simulink model "Nodal_Analysis"  (R2024b)
settings: Solver=VariableStepAuto  StartTime=0.0  StopTime=10.0  RelTol=1e-3
libraries: spsSeriesRLCBranchLib x15, spsVoltageMeasurementLib x13, spsDCVoltageSourceLib x5, spsACVoltageSourceLib x2, spsCurrentMeasurementLib x1, spsControlledCurrentSourceLib x1, sps_lib x1
settings Model: Creator=priya  LastModifiedBy=priya

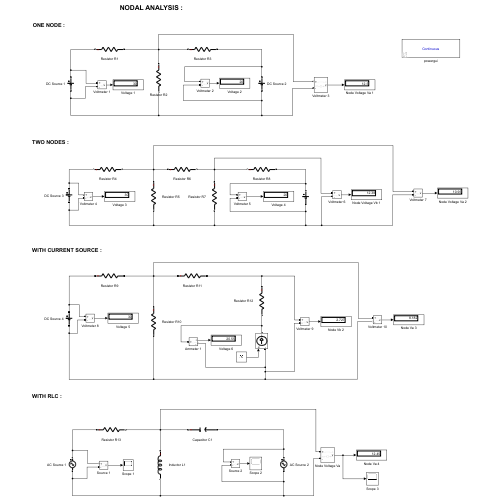
[thumbnail: Simulink's stored preview of the top-level diagram]
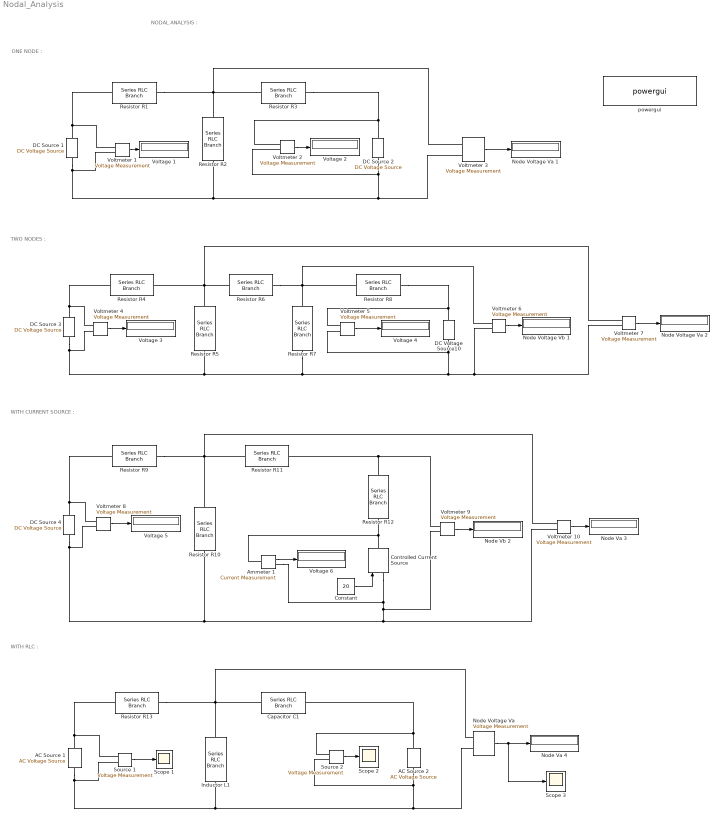
== system Nodal_Analysis ==
  note: WITH CURRENT SOURCE :
  note: TWO NODES :
  note: ONE NODE :
  note: NODAL ANALYSIS :
  note: WITH RLC :
  AC Source 1 : spsACVoltageSourceLib/AC Voltage Source  Amplitude=30  Phase=0  Frequency=60  SampleTime=0  Measurements=None  BusType=swing  Pref=10e3  Qref=0  Qmin=-inf  Qmax=+inf
  AC Source 2 : spsACVoltageSourceLib/AC Voltage Source  Amplitude=20  Phase=0  Frequency=60  SampleTime=0  Measurements=None  BusType=swing  Pref=10e3  Qref=0  Qmin=-inf  Qmax=+inf
  Ammeter 1 : spsCurrentMeasurementLib/Current Measurement  PhasorSimulation=off  OutputType=Complex  PSBequivalent=0
  Capacitor C1 : spsSeriesRLCBranchLib/Series RLC Branch  LConnTagsString=__new0  RConnTagsString=__new0  BranchType=C  Resistance=10  Inductance=1e-3  SetiL0=off  InitialCurrent=0  Capacitance=106.1e-6  Setx0=off  InitialVoltage=0  Measurements=None
  Constant : Constant  Value=20
  Controlled Current Source : spsControlledCurrentSourceLib/Controlled Current Source  Initialize=on  Source_Type=DC  Amplitude=20  Phase=0  Frequency=0  Measurements=None
  DC Source 1 : spsDCVoltageSourceLib/DC Voltage Source  Amplitude=30  Measurements=None
  DC Source 2 : spsDCVoltageSourceLib/DC Voltage Source  Amplitude=20  Measurements=None
  DC Source 3 : spsDCVoltageSourceLib/DC Voltage Source  Amplitude=30  Measurements=None
  DC Source 4 : spsDCVoltageSourceLib/DC Voltage Source  Amplitude=30  Measurements=None
  DC Voltage Source10 : spsDCVoltageSourceLib/DC Voltage Source  Amplitude=20  Measurements=None
  Inductor L1 : spsSeriesRLCBranchLib/Series RLC Branch  LConnTagsString=__new0  RConnTagsString=__new0  BranchType=L  Resistance=5  Inductance=0.01  SetiL0=off  InitialCurrent=0  Capacitance=1e-6  Setx0=off  InitialVoltage=0  Measurements=None
  Node Va 3 : Display
  Node Va 4 : Display
  Node Vb 2 : Display
  Node Voltage Va : spsVoltageMeasurementLib/Voltage Measurement  PhasorSimulation=off  OutputType=Complex  PSBequivalent=0
  Node Voltage Va 1 : Display
  Node Voltage Va 2 : Display
  Node Voltage Vb 1 : Display
  Resistor R{1,3..4,7,9,11,13} (7 alike) : spsSeriesRLCBranchLib/Series RLC Branch  LConnTagsString=__new0  RConnTagsString=__new0  BranchType=R  Resistance=10  Inductance=1e-3  SetiL0=off  InitialCurrent=0  Capacitance=1e-6  Setx0=off  InitialVoltage=0  Measurements=None
  Resistor R{2,5..6,8,10,12} (6 alike) : spsSeriesRLCBranchLib/Series RLC Branch  LConnTagsString=__new0  RConnTagsString=__new0  BranchType=R  Resistance=5  Inductance=1e-3  SetiL0=off  InitialCurrent=0  Capacitance=1e-6  Setx0=off  InitialVoltage=0  Measurements=None
  Scope 1 : Scope
  Scope 2 : Scope
  Scope 3 : Scope
  Source 1 : spsVoltageMeasurementLib/Voltage Measurement  PhasorSimulation=off  OutputType=Complex  PSBequivalent=0
  Source 2 : spsVoltageMeasurementLib/Voltage Measurement  PhasorSimulation=off  OutputType=Complex  PSBequivalent=0
  Voltage {1..6} (6 alike) : Display
  Voltmeter {1..10} (10 alike) : spsVoltageMeasurementLib/Voltage Measurement  PhasorSimulation=off  OutputType=Complex  PSBequivalent=0
  powergui : sps_lib/powergui  Priority=1  SimulationMode=Continuous  SampleTime=50e-6  frequency=60  Iterations=50  frequencyindice=0  Pbase=100e6  ErrMax=1e-4  UnitsV=kV  UnitsW=MW  buscounter=0  FunctionMessages=off  echomessages=off  EnableUseOfTLC=off  CurrentSourceSwitches=off  DisableSnubberDevices=off  DisableRonSwitches=off  DisableVfSwitches=off  DisplayEquations=off  AutomaticDiscreteSolvers=off  SolverType=Tustin/Backward Euler (TBE)  Interpol=off  ExternalGateDelay=off  methode=off  Ts=100  x0status=blocks  SPID=on  SwTol=0  HookPort=off  NonlinearTolerance=1e-4  nMaxIteration=100  ContinueOnMaxIteration=off  RestoreLinks=warning  ResistiveCurrentMeasurement=off  Frange=[0:2:500]  Ylog=off  Xlog=on  ShowGrid=off  save=off  variable=ZData  structure=0  ZoomFFT=off  StartTime=0.0  cycles=1  DisplayStyle=1  fundamental=60  FreqAxis=off  MaxFrequency=1000  frequencyindicesteady=1  RmsSteady=1  display=off
  wires:
  Voltmeter 1/1 -> Voltage 1/1
  Voltmeter 2/1 -> Voltage 2/1
  Voltmeter 3/1 -> Node Voltage Va 1/1
  Voltmeter 4/1 -> Voltage 3/1
  Voltmeter 5/1 -> Voltage 4/1
  Voltmeter 6/1 -> Node Voltage Vb 1/1
  Voltmeter 7/1 -> Node Voltage Va 2/1
  Voltmeter 8/1 -> Voltage 5/1
  Voltmeter 9/1 -> Node Vb 2/1
  Voltmeter 10/1 -> Node Va 3/1
  Constant/1 -> Controlled Current Source/1
  Ammeter 1/1 -> Voltage 6/1
  Source 1/1 -> Scope 1/1
  Node Voltage Va/1 -> Scope 3/1, Node Va 4/1
  Source 2/1 -> Scope 2/1
  connections:
  DC Source 1/RConn1 -- Resistor R1/LConn1 -- Voltmeter 1/LConn1
  Resistor R1/RConn1 -- Resistor R2/LConn1 -- Voltmeter 3/LConn1 -- Resistor R3/LConn1
  DC Source 1/LConn1 -- Voltmeter 3/LConn2 -- Voltmeter 2/LConn2 -- DC Source 2/LConn1 -- Resistor R2/RConn1 -- Voltmeter 1/LConn2
  Resistor R3/RConn1 -- Voltmeter 2/LConn1 -- DC Source 2/RConn1
  DC Source 3/RConn1 -- Resistor R4/LConn1 -- Voltmeter 4/LConn1
  DC Source 3/LConn1 -- Voltmeter 4/LConn2 -- Voltmeter 7/LConn2 -- Voltmeter 6/LConn2 -- DC Voltage Source10/LConn1 -- Voltmeter 5/LConn2 -- Resistor R7/RConn1 -- Resistor R5/RConn1
  Resistor R6/LConn1 -- Resistor R5/LConn1 -- Voltmeter 7/LConn1 -- Resistor R4/RConn1
  Resistor R6/RConn1 -- Resistor R7/LConn1 -- Voltmeter 6/LConn1 -- Resistor R8/LConn1
  Resistor R8/RConn1 -- Voltmeter 5/LConn1 -- DC Voltage Source10/RConn1
  Resistor R9/LConn1 -- Voltmeter 8/LConn1 -- DC Source 4/RConn1
  Resistor R9/RConn1 -- Resistor R10/LConn1 -- Voltmeter 10/LConn1 -- Resistor R11/LConn1
  DC Source 4/LConn1 -- Voltmeter 10/LConn2 -- Voltmeter 9/LConn2 -- Controlled Current Source/LConn1 -- Ammeter 1/RConn1 -- Resistor R10/RConn1 -- Voltmeter 8/LConn2
  Voltmeter 9/LConn1 -- Resistor R12/LConn1 -- Resistor R11/RConn1
  Controlled Current Source/RConn1 -- Ammeter 1/LConn1 -- Resistor R12/RConn1
  Source 1/LConn2 -- Source 2/LConn2 -- AC Source 2/LConn1 -- Node Voltage Va/LConn2 -- Inductor L1/RConn1 -- AC Source 1/LConn1
  Inductor L1/LConn1 -- Capacitor C1/LConn1 -- Resistor R13/RConn1 -- Node Voltage Va/LConn1
  Source 1/LConn1 -- Resistor R13/LConn1 -- AC Source 1/RConn1
  AC Source 2/RConn1 -- Capacitor C1/RConn1 -- Source 2/LConn1
